simulink model "N3_TE0722A4"  (R2013b)
settings: Solver=ode45  StartTime=0.0  StopTime=1e-4  RelTol=1e-3
PreLoadFcn:
  | fpgaclk=1/32.768e6
  | SerialData=[1,zeros(1,11),1,0,0,1]
  | load ../window
  | win=win'   %Go back to using flatter and wider windowed sync function
  | %load ../hanning    %use Hahn window
  | 
  | load ../PREemphasis   %For pre-empasis and deemphasis FIRs
  | 
  | LUT3=xls2LUT2('../IQI_Qdemod.xls')
  | load ../FIRiq2
  | % xls2LUT
  | 
  | GetProgFiles
  | 
  | PinAssignments    %Get Pin references for TE0722
  | 
  | 
  | 
  | 
  | 
  | %LCD
  | LCDdata=[LCD_D7,LCD_D6,LCD_D5,LCD_D4,LCD_D3,LCD_D2,LCD_D1,LCD_D0] %Note MSB...LSB!
  | LCDctrl=[LCD_E,LCD_RW,LCD_RS];
  | 
  | %for RS232 on pins 3 and 5 of USBB
  | 
  | %BT chip connections for WT12
  | 
  | RX_BT=RXD
  | TX_BT=TXD
  | 
  | RST_BB=RES
  | 
  | %PCMC=PCMC
  | %PCMS=PCMS
  | %PCMI=PCMI
  | %PCMO=PCMO
  | 
  | %Aliases:
  | SRDBT=PCMI
  | STDBT=PCMO
  | SCLK_BT=PCMC
  | SFS_BT=PCMS
  | 
  | %ADC control
  | 
  | %SDOA=SDOA
  | %SDOB=SDOB
  | %SCK=SCK
  | CONV=Csbar
  | CAL=Cal
  | 
  | ADC_G=[ADC_G3,ADC_G2,ADC_G1,ADC_G0]
  | %PD settings hard coded now
  | 
  | %%%%%%
  | TX_LOW=TX_Low
  | 
  | %Leds
  | %Defined inPinassignments
  | ... (+8 lines)
StartFcn:
  | fpgaclk=1/32.768e6
  | SerialData=[1,zeros(1,11),1,0,0,1]
values from neighbouring files (symbols this model uses):
  ADC_G0 = {'P10'}    [PinAssignments.m]
  ADC_G1 = {'P11'}    [PinAssignments.m]
  ADC_G2 = {'N14'}    [PinAssignments.m]
  ADC_G3 = {'M11'}    [PinAssignments.m]
  Cal = {'L12'}    [PinAssignments.m]
  Csbar = {'M12'}    [PinAssignments.m]
  LCD_D0 = {'J13'}    [PinAssignments.m]
  LCD_D1 = {'J14'}    [PinAssignments.m]
  LCD_D2 = {'F15'}    [PinAssignments.m]
  LCD_D3 = {'H14'}    [PinAssignments.m]
  LCD_D4 = {'G12'}    [PinAssignments.m]
  LCD_D5 = {'L15'}    [PinAssignments.m]
  LCD_D6 = {'M14'}    [PinAssignments.m]
  LCD_D7 = {'K15'}    [PinAssignments.m]
  PCMC = {'H11'}    [PinAssignments.m]
  PCMI = {'H12'}    [PinAssignments.m]
  PCMO = {'N13'}    [PinAssignments.m]
  PCMS = {'M10'}    [PinAssignments.m]
  RES = {'G11'}    [PinAssignments.m]
  RXD = {'H13'}    [PinAssignments.m]
  TX_Low = {'P15'}    [PinAssignments.m]
  TXD = {'P13'}    [PinAssignments.m]
undefined symbols (not defined in the file or in its folder): FIRRX, FIRTX
libraries: xbsIndex_r4 x1100, MyFunctions x42
(part 2 of 9)

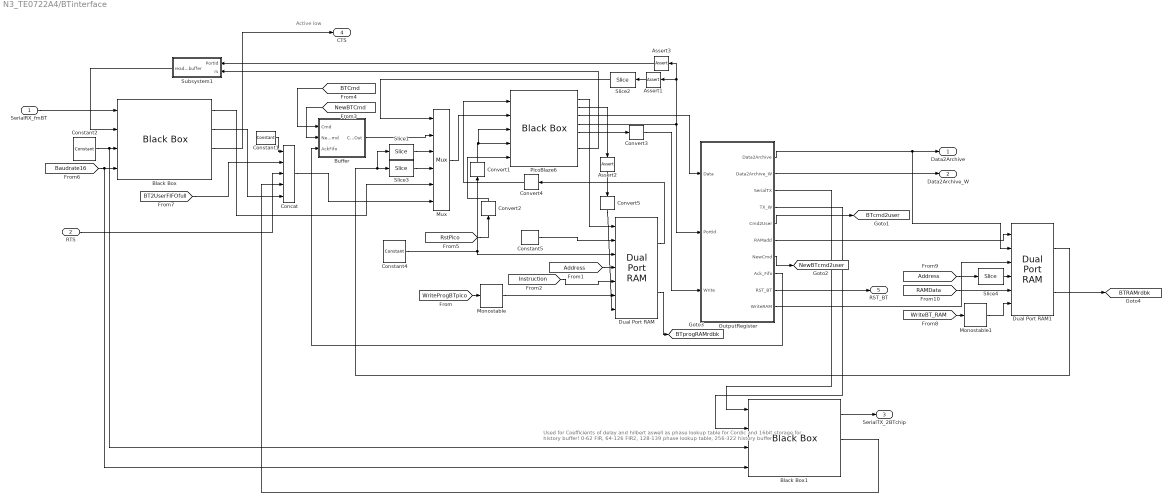
== system N3_TE0722A4/BTinterface ==
  note: Used for Coefficients of delay and hilbert aswell as phase lookup table for Cordic and 16bit storage for history buffer!
      | 0-62 FIR, 64-126 FIR2, 128-139 phase lookup table, 256-322 history buffer
  note: Active low
  SerialRX_fmBT : Inport
  RTS : Inport  Port=2
  Assert1 : xbsIndex_r4/Assert  assert_type=off  type_source=Explicitly  gui_display_data_type=Fixed-point  arith_type="Signed  (2's comp)"  n_bits=16  bin_pt=14  preci_type=Single  exp_width=8  frac_width=24  assert_rate=on  rate_source=Explicitly  period=fpgaclk  output_port=on  block_type=assert
  Assert2 : xbsIndex_r4/Assert  assert_type=off  type_source=Explicitly  gui_display_data_type=Fixed-point  arith_type="Signed  (2's comp)"  n_bits=16  bin_pt=14  preci_type=Single  exp_width=8  frac_width=24  assert_rate=on  rate_source=Explicitly  period=fpgaclk  output_port=on  block_type=assert
  Assert3 : xbsIndex_r4/Assert  assert_type=off  type_source=Explicitly  gui_display_data_type=Fixed-point  arith_type="Signed  (2's comp)"  n_bits=16  bin_pt=14  preci_type=Single  exp_width=8  frac_width=24  assert_rate=on  rate_source=Explicitly  period=fpgaclk  output_port=on  block_type=assert
  Black Box : xbsIndex_r4/Black Box  init_code=uart_rxce_config  sim_method=Inactive  verbose=off  block_type=blackbox2
      settings: block_version=8.2.02
  Black Box1 : xbsIndex_r4/Black Box  init_code=uart_txce_config  sim_method=Inactive  verbose=off  block_type=blackbox2
      settings: infoedit="Incorporates black box HDL and simulation model into a System Generator design.<P><P>You must supply a Black Box with certain information about the HDL component you would like to bring into System Generator. This information is provided through a Matlab function.<P><P>When \"Simulation mode\" is set to \"Inactive\", you will typically want to provide a separate simulation model by using a Simulation Multiplexer.<P>When \"Simulation mode\" is set to \"External co-simulator\", you must include a ModelSim block in the design."  block_version=8.2.02
  Buffer : Subsystem
  Concat : xbsIndex_r4/Concat  num_inputs=5  dbl_ovrd=off  block_type=concat
      settings: block_version=VER_STRING_GOES_HERE
  Constant1 : xbsIndex_r4/Constant  const=0  gui_display_data_type=Fixed-point  arith_type=Unsigned  n_bits=4  bin_pt=0  preci_type=Single  exp_width=8  frac_width=24  explicit_period=on  period=fpgaclk  equ=P=C  opselect=C  inp2=PCIN>>17  opr=+  inp1=P  carry=CIN  dbl_ovrd=off  block_type=constant
      settings: block_version=VER_STRING_GOES_HERE
  Constant2 : xbsIndex_r4/Constant  const=0  gui_display_data_type=Fixed-point  arith_type=Unsigned  n_bits=1  bin_pt=0  preci_type=Single  exp_width=8  frac_width=24  explicit_period=on  period=fpgaclk  equ=P=C  opselect=C  inp2=PCIN>>17  opr=+  inp1=P  carry=CIN  dbl_ovrd=off  block_type=constant
      settings: block_version=VER_STRING_GOES_HERE
  Constant4 : xbsIndex_r4/Constant  const=0  gui_display_data_type=Fixed-point  arith_type=Boolean  n_bits=1  bin_pt=0  preci_type=Single  exp_width=8  frac_width=24  explicit_period=on  period=fpgaclk  equ=P=C  opselect=C  inp2=PCIN>>17  opr=+  inp1=P  carry=CIN  dbl_ovrd=off  block_type=constant
      settings: block_version=VER_STRING_GOES_HERE
  Constant5 : xbsIndex_r4/Constant  const=0  gui_display_data_type=Fixed-point  arith_type=Unsigned  n_bits=18  bin_pt=0  preci_type=Single  exp_width=8  frac_width=24  explicit_period=on  period=fpgaclk  equ=P=C  opselect=C  inp2=PCIN>>17  opr=+  inp1=P  carry=CIN  dbl_ovrd=off  block_type=constant
      settings: block_version=VER_STRING_GOES_HERE
  Convert1 : xbsIndex_r4/Convert  gui_display_data_type=Fixed-point  arith_type=Boolean  n_bits=16  bin_pt=0  float_type=Single  exp_bits=8  fraction_bits=24  quantization=Truncate  overflow=Wrap  en=off  latency=0  pipeline=off  dbl_ovrd=off  block_type=convert
      settings: xl_area=[0 0 0 0 0 0 0]  block_version=VER_STRING_GOES_HERE
  Convert2 : xbsIndex_r4/Convert  gui_display_data_type=Fixed-point  arith_type=Boolean  n_bits=16  bin_pt=0  float_type=Single  exp_bits=8  fraction_bits=24  quantization=Truncate  overflow=Wrap  en=off  latency=0  pipeline=off  dbl_ovrd=off  block_type=convert
      settings: xl_area=[0, 0, 0, 0, 0, 0, 0]  block_version=VER_STRING_GOES_HERE
  Convert3 : xbsIndex_r4/Convert  gui_display_data_type=Fixed-point  arith_type=Boolean  n_bits=16  bin_pt=0  float_type=Single  exp_bits=8  fraction_bits=24  quantization=Truncate  overflow=Wrap  en=off  latency=0  pipeline=off  dbl_ovrd=off  block_type=convert
      settings: xl_area=[0 0 0 0 0 0 0]  block_version=VER_STRING_GOES_HERE
  Convert4 : xbsIndex_r4/Convert  gui_display_data_type=Fixed-point  arith_type=Unsigned  n_bits=18  bin_pt=0  float_type=Single  exp_bits=8  fraction_bits=24  quantization=Truncate  overflow=Wrap  en=off  latency=0  pipeline=off  dbl_ovrd=off  block_type=convert
      settings: xl_area=[0, 0, 0, 0, 0, 0, 0]  block_version=VER_STRING_GOES_HERE
  Convert5 : xbsIndex_r4/Convert  gui_display_data_type=Boolean  arith_type=Boolean  n_bits=18  bin_pt=0  float_type=Single  exp_bits=8  fraction_bits=24  quantization=Truncate  overflow=Wrap  en=off  latency=0  pipeline=off  dbl_ovrd=off  block_type=convert
      settings: xl_area=[0, 0, 0, 0, 0, 0, 0]  block_version=VER_STRING_GOES_HERE
  Dual Port RAM : xbsIndex_r4/Dual Port RAM  depth=1024*4  initVector=BTprog  distributed_mem=Block RAM  init_a=0  init_b=0  rst_a=off  rst_b=off  en_a=on  en_b=off  latency=1  write_mode_A=Read After Write  write_mode_B=Read After Write  optimize=Area  dbl_ovrd=off  block_type=dpram
      settings: block_version=8.2.02
  Dual Port RAM1 : xbsIndex_r4/Dual Port RAM  depth=1024  initVector=BTmessages  distributed_mem=Block RAM  init_a=0  init_b=0  rst_a=off  rst_b=off  en_a=off  en_b=off  latency=1  write_mode_A=Read After Write  write_mode_B=Read After Write  optimize=Area  dbl_ovrd=off  block_type=dpram
      settings: block_version=8.2.02
  Monostable : MyFunctions/Monostable
  Monostable1 : MyFunctions/Monostable
  Mux : xbsIndex_r4/Mux  inputs=5  en=off  latency=1  precision=Full  arith_type=Unsigned  n_bits=16  bin_pt=14  quantization=Truncate  overflow=Wrap  dbl_ovrd=off  block_type=mux
      settings: xl_area=[16 0 0 32 0 0 0]  block_version=VER_STRING_GOES_HERE
  OutputRegister : Subsystem
  PicoBlaze6 : xbsIndex_r4/Black Box  init_code=kcpsm6_CE_256_4k_config  sim_method=Inactive  verbose=off  block_type=blackbox2
  Slice1 : xbsIndex_r4/Slice  nbits=8  boolean_output=off  mode=Lower Bit Location + Width  bit1=0  base1=MSB of Input  bit0=8  base0=LSB of Input  dbl_ovrd=off  block_type=slice
      settings: block_version=VER_STRING_GOES_HERE
  Slice2 : xbsIndex_r4/Slice  nbits=3  boolean_output=off  mode=Lower Bit Location + Width  bit1=0  base1=MSB of Input  bit0=0  base0=LSB of Input  dbl_ovrd=off  block_type=slice
      settings: block_version=VER_STRING_GOES_HERE
  Slice3 : xbsIndex_r4/Slice  nbits=8  boolean_output=off  mode=Lower Bit Location + Width  bit1=0  base1=MSB of Input  bit0=0  base0=LSB of Input  dbl_ovrd=off  block_type=slice
      settings: block_version=VER_STRING_GOES_HERE
  Slice4 : xbsIndex_r4/Slice  nbits=10  boolean_output=off  mode=Lower Bit Location + Width  bit1=0  base1=MSB of Input  bit0=0  base0=LSB of Input  dbl_ovrd=off  block_type=slice
      settings: block_version=VER_STRING_GOES_HERE
  Subsystem1 : Subsystem
  Data2Archive : Outport
  Data2Archive_W : Outport  Port=2
  SerialTX_2BTchip : Outport  Port=3
  CTS : Outport  Port=4
  RST_BT : Outport  Port=5
  tag scope: BTRAMrdbk=global, BTcmd2user=global, BTprogRAMrdbk=global, NewBTcmd2user=global
  wires:
  Convert4/1 -> PicoBlaze6/1
  [RstPico] -> Convert2/1
  PicoBlaze6/5 -> Convert3/1
  PicoBlaze6/4 -> Assert1/1, Assert3/1, OutputRegister/2(PortId)
  PicoBlaze6/3 -> OutputRegister/1(Data)
  PicoBlaze6/1 -> Dual Port RAM/1
  Convert2/1 -> PicoBlaze6/5
  Mux/1 -> PicoBlaze6/2
  Dual Port RAM/1 -> Convert4/1
  Constant4/1 -> Dual Port RAM/3, Convert1/1
  Constant5/1 -> Dual Port RAM/2
  Slice2/1 -> Mux/1
  Convert1/1 -> PicoBlaze6/3, PicoBlaze6/4
  OutputRegister/5(Cmd2User) -> [BTcmd2user]
  OutputRegister/8(Ack_Fifo) -> Buffer/3(AckFifo)
  Convert3/1 -> OutputRegister/3(Write)
  OutputRegister/1(Data2Archive) -> Data2Archive/1, Dual Port RAM1/2
  [Address] -> Dual Port RAM/4
  Buffer/1(CmdOut) -> Mux/2
  [Instruction] -> Dual Port RAM/5
  OutputRegister/7(NewCmd) -> [NewBTcmd2user]
  [BTCmd] -> Buffer/1(Cmd)
  [NewBTCmd] -> Buffer/2(NewCmd)
  Black Box/1 -> Mux/5
  Subsystem1/1(read_buffer) -> Black Box/2
  Constant1/1 -> Concat/1
  PicoBlaze6/7 -> Subsystem1/2(rs)
  Black Box1/1 -> SerialTX_2BTchip/1
  Black Box/2 -> Concat/5
  Concat/1 -> Mux/6
  SerialRX_fmBT/1 -> Black Box/1
  RTS/1 -> Concat/3
  Black Box/3 -> CTS/1
  OutputRegister/3(SerialTX) -> Black Box1/1
  OutputRegister/4(TX_W) -> Black Box1/2
  [Baudrate16] -> Black Box/4, Black Box1/4
  OutputRegister/2(Data2Archive_W) -> Data2Archive_W/1
  OutputRegister/9(RST_BT) -> RST_BT/1
  Monostable/1 -> Dual Port RAM/6
  Constant2/1 -> Black Box/3, Black Box1/3
  [BT2UserFIFOfull] -> Concat/2
  Black Box1/2 -> Concat/4
  [WriteProgBTpico] -> Monostable/1
  Dual Port RAM/2 -> [BTprogRAMrdbk]
  [Address] -> Slice4/1
  [RAMData] -> Dual Port RAM1/5
  Monostable1/1 -> Dual Port RAM1/6
  [WriteBT_RAM] -> Monostable1/1
  Dual Port RAM1/2 -> [BTRAMrdbk]
  OutputRegister/6(RAMadd) -> Dual Port RAM1/1
  Slice1/1 -> Mux/3
  Slice3/1 -> Mux/4
  Dual Port RAM1/1 -> Slice1/1, Slice3/1
  OutputRegister/10(WriteRAM) -> Dual Port RAM1/3
  Slice4/1 -> Dual Port RAM1/4
  PicoBlaze6/2 -> Assert2/1
  Assert3/1 -> Subsystem1/1(PortId)
  Assert1/1 -> Slice2/1
  Assert2/1 -> Convert5/1
  Convert5/1 -> Dual Port RAM/7

== system N3_TE0722A4/Bit_Corrector ==
  note: Does the sign extnsion
  In1 : Inport
  Concat : xbsIndex_r4/Concat  num_inputs=3  dbl_ovrd=off  block_type=concat
      settings: block_version=12.2
  Reinterpret : xbsIndex_r4/Reinterpret  force_arith_type=on  arith_type="Signed  (2's comp)"  force_bin_pt=on  bin_pt=15  block_type=reinterpret
      settings: infoedit="Changes signal type without altering the binary representation.   You can changed the signal between signed and unsigned, and relocate the binary point.<br><br>Hardware notes: In hardware this block costs nothing.<br><br>Example:  Suppose the input is 6 bits wide, signed, with 2 fractional bits, and the output is forced to unsigned with 0 fractional bits.  Then an input of -2.0 (1110.00 in binary 2's complement) becomes an output of 56 (111000 in binary)."  block_version=8.2.02
  Slice : xbsIndex_r4/Slice  nbits=14  boolean_output=off  mode=Lower Bit Location + Width  bit1=0  base1=MSB of Input  bit0=0  base0=LSB of Input  dbl_ovrd=off  block_type=slice
      settings: block_version=12.2
  Slice1 : xbsIndex_r4/Slice  nbits=1  boolean_output=off  mode=Lower Bit Location + Width  bit1=0  base1=MSB of Input  bit0=13  base0=LSB of Input  dbl_ovrd=off  block_type=slice
      settings: block_version=12.2
  Slice2 : xbsIndex_r4/Slice  nbits=1  boolean_output=off  mode=Lower Bit Location + Width  bit1=0  base1=MSB of Input  bit0=13  base0=LSB of Input  dbl_ovrd=off  block_type=slice
      settings: block_version=12.2
  Out1 : Outport
  wires:
  In1/1 -> Slice2/1, Slice1/1, Slice/1
  Slice2/1 -> Concat/1
  Slice1/1 -> Concat/2
  Slice/1 -> Concat/3
  Concat/1 -> Reinterpret/1
  Reinterpret/1 -> Out1/1

== system N3_TE0722A4/Bit_Corrector1 ==
  note: Does the sign extnsion
  In1 : Inport
  Concat : xbsIndex_r4/Concat  num_inputs=3  dbl_ovrd=off  block_type=concat
      settings: block_version=12.2
  Reinterpret : xbsIndex_r4/Reinterpret  force_arith_type=on  arith_type="Signed  (2's comp)"  force_bin_pt=on  bin_pt=15  block_type=reinterpret
      settings: infoedit="Changes signal type without altering the binary representation.   You can changed the signal between signed and unsigned, and relocate the binary point.<br><br>Hardware notes: In hardware this block costs nothing.<br><br>Example:  Suppose the input is 6 bits wide, signed, with 2 fractional bits, and the output is forced to unsigned with 0 fractional bits.  Then an input of -2.0 (1110.00 in binary 2's complement) becomes an output of 56 (111000 in binary)."  block_version=8.2.02
  Slice : xbsIndex_r4/Slice  nbits=14  boolean_output=off  mode=Lower Bit Location + Width  bit1=0  base1=MSB of Input  bit0=0  base0=LSB of Input  dbl_ovrd=off  block_type=slice
      settings: block_version=12.2
  Slice1 : xbsIndex_r4/Slice  nbits=1  boolean_output=off  mode=Lower Bit Location + Width  bit1=0  base1=MSB of Input  bit0=13  base0=LSB of Input  dbl_ovrd=off  block_type=slice
      settings: block_version=12.2
  Slice2 : xbsIndex_r4/Slice  nbits=1  boolean_output=off  mode=Lower Bit Location + Width  bit1=0  base1=MSB of Input  bit0=13  base0=LSB of Input  dbl_ovrd=off  block_type=slice
      settings: block_version=12.2
  Out1 : Outport
  wires:
  In1/1 -> Slice2/1, Slice1/1, Slice/1
  Slice2/1 -> Concat/1
  Slice1/1 -> Concat/2
  Slice/1 -> Concat/3
  Concat/1 -> Reinterpret/1
  Reinterpret/1 -> Out1/1

== system N3_TE0722A4/ConstantDetect ==
  note: Pulses every 8 pulses of the 8kHz strobe ie at 1kHz
  Signal : Inport
  Strobe : Inport  Port=2
  Constant1 : xbsIndex_r4/Constant  const=4  gui_display_data_type=Fixed-point  arith_type=Unsigned  n_bits=4  bin_pt=0  preci_type=Single  exp_width=8  frac_width=24  explicit_period=off  period=1  equ=P=C  opselect=C  inp2=PCIN>>17  opr=+  inp1=P  carry=CIN  dbl_ovrd=off  block_type=constant
      settings: block_version=12.2
  Convert : xbsIndex_r4/Convert  gui_display_data_type=Fixed-point  arith_type=Boolean  n_bits=16  bin_pt=14  float_type=Single  exp_bits=8  fraction_bits=24  quantization=Truncate  overflow=Wrap  en=off  latency=0  pipeline=off  dbl_ovrd=off  block_type=convert
      settings: block_version=12.2
  Counter : xbsIndex_r4/Counter  cnt_type=Free Running  cnt_to=Inf  operation=Up  start_count=0  cnt_by_val=1  arith_type=Unsigned  n_bits=3  bin_pt=0  load_pin=off  rst=off  en=on  explicit_period=on  period=fpgaclk  use_behavioral_HDL=off  implementation=Fabric  dbl_ovrd=off  block_type=counter
      settings: block_version=12.2
  Counter1 : xbsIndex_r4/Counter  cnt_type=Free Running  cnt_to=Inf  operation=Up  start_count=0  cnt_by_val=1  arith_type=Unsigned  n_bits=4  bin_pt=0  load_pin=off  rst=on  en=on  explicit_period=on  period=fpgaclk  use_behavioral_HDL=off  implementation=Fabric  dbl_ovrd=off  block_type=counter
      settings: block_version=12.2
  Delay : xbsIndex_r4/Delay  rst=off  infoeditControl=Selection of Reset will increase slice count due to use of real FFs and instead of SRLs  en=on  latency=1  reg_retiming=off  dbl_ovrd=off  block_type=delay
      settings: block_version=12.2
  Delay1 : xbsIndex_r4/Delay  rst=off  infoeditControl=Selection of Reset will increase slice count due to use of real FFs and instead of SRLs  en=on  latency=1  reg_retiming=off  dbl_ovrd=off  block_type=delay
      settings: block_version=12.2
  Logical : xbsIndex_r4/Logical  logical_function=AND  inputs=2  en=off  latency=0  precision=Full  arith_type=Unsigned  n_bits=16  bin_pt=0  align_bp=on  dbl_ovrd=off  block_type=logical
      settings: block_version=12.2
  Monostable : MyFunctions/Monostable
  Register : xbsIndex_r4/Register  init=0  rst=off  en=on  dbl_ovrd=off  block_type=register
      settings: block_version=12.2
  Relational : xbsIndex_r4/Relational  mode=a=b  op_type=Bool  en=off  latency=1  dbl_ovrd=off  block_type=relational
      settings: block_version=12.2
  Relational1 : xbsIndex_r4/Relational  mode=a<b  op_type=Bool  en=off  latency=1  dbl_ovrd=off  block_type=relational
      settings: block_version=12.2
  Slice : xbsIndex_r4/Slice  nbits=1  boolean_output=off  mode=Upper Bit Location + Width  bit1=0  base1=MSB of Input  bit0=0  base0=LSB of Input  dbl_ovrd=off  block_type=slice
      settings: block_version=12.2
  IsConstant : Outport
  wires:
  Signal/1 -> Delay/1
  Strobe/1 -> Delay/2, Delay1/2, Counter/1, Logical/2
  Counter/1 -> Slice/1
  Slice/1 -> Convert/1
  Convert/1 -> Monostable/1
  Monostable/1 -> Counter1/1, Register/2
  Counter1/1 -> Register/1
  Constant1/1 -> Relational1/1
  Register/1 -> Relational1/2
  Relational1/1 -> IsConstant/1
  Relational/1 -> Logical/1
  Logical/1 -> Counter1/2
  Delay/1 -> Delay1/1, Relational/1
  Delay1/1 -> Relational/2

== system N3_TE0722A4/DAC (XAPP154) ==
  note: This subsystem implements a delta-sigma DAC
  note: The 'Delta Adder' computes the difference
      | between the current DAC input and the current
      | DAC output.  The two concatenators create
      | a 16-bit output with the DAC output copied in the
      | two MSB positions. This effectively creates a
      | difference from the 'Delta Adder' when the DAC
      | output is 1.
  note: The 'Sigma Adder' accumulates the
      | differences produced by the 'Delta Adder'
      | by using 'r1' to storing the adder output on
      | each succesive cycle.  The MSB of the 'r1'
      | output is sliced off and provides the DAC
      | output.
  note: The pulse string is registered before
      | it is driven on the DAC output port.
  note: Constants sampled at 40*fpgaclk
      | to reduce modulation frequency
  DAC_In : Inport
  Disable_Audio : Inport  Port=2
  Concat : xbsIndex_r4/Concat  num_inputs=2  dbl_ovrd=off  block_type=concat
      settings: block_version=VER_STRING_GOES_HERE
  Concat1 : xbsIndex_r4/Concat  num_inputs=2  dbl_ovrd=off  block_type=concat
      settings: block_version=VER_STRING_GOES_HERE
  Constant : xbsIndex_r4/Constant  const=0  gui_display_data_type=Fixed-point  arith_type=Boolean  n_bits=1  bin_pt=0  preci_type=Single  exp_width=8  frac_width=24  explicit_period=on  period=fpgaclk*40  equ=P=C  opselect=C  inp2=PCIN>>17  opr=+  inp1=P  carry=CIN  dbl_ovrd=off  block_type=constant
      settings: block_version=VER_STRING_GOES_HERE
  Constant2 : xbsIndex_r4/Constant  const=0  gui_display_data_type=Fixed-point  arith_type=Unsigned  n_bits=14  bin_pt=0  preci_type=Single  exp_width=8  frac_width=24  explicit_period=on  period=fpgaclk*40  equ=P=C  opselect=C  inp2=PCIN>>17  opr=+  inp1=P  carry=CIN  dbl_ovrd=off  block_type=constant
      settings: block_version=VER_STRING_GOES_HERE
  Delta Adder : xbsIndex_r4/AddSub  mode=Addition  use_carryin=off  use_carryout=off  en=on  latency=1  precision=User Defined  arith_type=Unsigned  n_bits=16  bin_pt=0  quantization=Truncate  overflow=Wrap  use_behavioral_HDL=on  hw_selection=Fabric  pipelined=off  use_rpm=off  dbl_ovrd=off  block_type=addsub
      settings: xl_area=[8 0 0 16 0 0 0]  block_version=VER_STRING_GOES_HERE
  Inverter : xbsIndex_r4/Inverter  en=off  latency=0  dbl_ovrd=off  block_type=inv
      settings: block_version=8.2.02
  Register1 : xbsIndex_r4/Register  init=0  rst=on  en=off  dbl_ovrd=off  block_type=register
      settings: xl_area=[1 1 0 0 0 0 0]  block_version=VER_STRING_GOES_HERE
  Sigma Adder : xbsIndex_r4/AddSub  mode=Addition  use_carryin=off  use_carryout=off  en=off  latency=0  precision=User Defined  arith_type=Unsigned  n_bits=16  bin_pt=0  quantization=Truncate  overflow=Wrap  use_behavioral_HDL=on  hw_selection=Fabric  pipelined=off  use_rpm=off  dbl_ovrd=off  block_type=addsub
      settings: xl_area=[8 0 0 16 0 0 0]  block_version=VER_STRING_GOES_HERE
  Slice1 : xbsIndex_r4/Slice  nbits=1  boolean_output=off  mode=Upper Bit Location + Width  bit1=0  base1=MSB of Input  bit0=0  base0=LSB of Input  dbl_ovrd=off  block_type=slice
      settings: infoedit="Extracts a given range of bits from each input sample and presents it at the output.  The output type is ordinarily unsigned with binary point at zero, but can be Boolean when the slice is one bit wide.<P><P>Hardware notes: In hardware this block costs nothing."  block_version=VER_STRING_GOES_HERE
  r1 : xbsIndex_r4/Register  init=2^6  rst=on  en=off  dbl_ovrd=off  block_type=register
      settings: xl_area=[8 16 0 0 0 0 0]  block_version=VER_STRING_GOES_HERE
  DAC_Out : Outport
  wires:
  DAC_In/1 -> Delta Adder/1
  Register1/1 -> DAC_Out/1
  r1/1 -> Slice1/1, Sigma Adder/1
  Sigma Adder/1 -> r1/1
  Constant/1 -> r1/2
  Concat1/1 -> Delta Adder/2
  Concat/1 -> Concat1/1
  Slice1/1 -> Register1/1, Concat/1, Concat/2
  Constant2/1 -> Concat1/2
  Delta Adder/1 -> Sigma Adder/2
  Disable_Audio/1 -> Register1/2, Inverter/1
  Inverter/1 -> Delta Adder/3

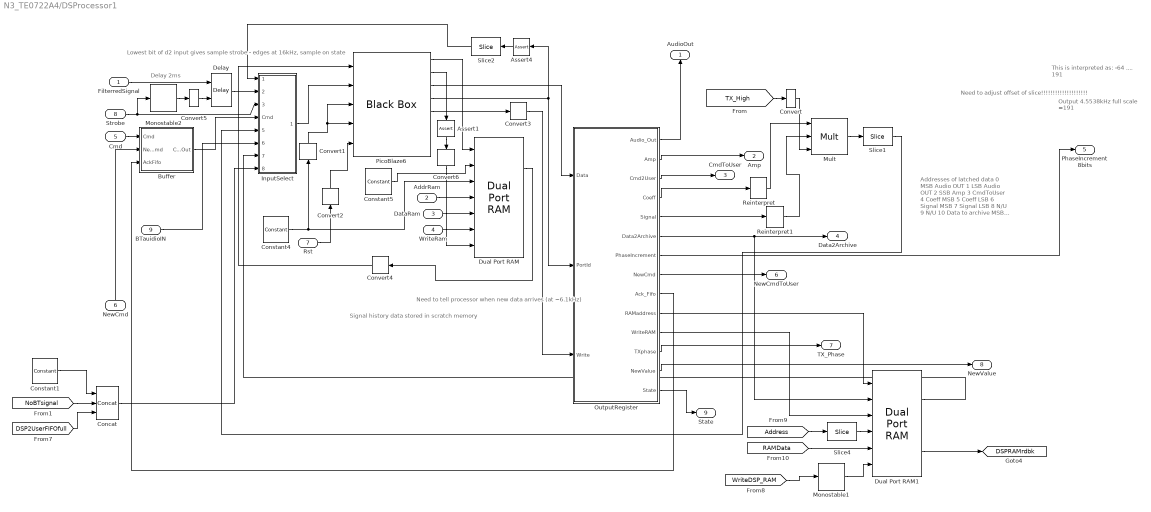
== system N3_TE0722A4/DSProcessor1 ==
  note: Need to adjust offset of slice!!!!!!!!!!!!!!!!!!!!
  note: Need to tell processor when new data arrives (at ~6.1kHz)
  note: Lowest bit of d2 input gives sample strobe - edges at 16kHz, sample on state
  note: Output 4.5538kHz
      | full scale =191
  note: This is interpreted as:
      | -64 .... 191
  note: Signal history data stored in scratch memory
  note: Addresses of latched data
      | 0 MSB Audio OUT
      | 1 LSB Audio OUT
      | 2 SSB Amp
      | 3 CmdToUser
      | 4 Coeff MSB
      | 5 Coeff LSB
      | 6 Signal MSB
      | 7 Signal LSB
      | 8 N/U
      | 9 N/U
      | 10 Data to archive MSB
      | 11 Data to archive LSB
      | 12 Control bits:
      | 	0
      | 	1
      | 	2
      | 	3
      | 	4
      | 	5 Ack Fifo
      |
      | 13 Audio Freq MSB
  note: Delay 2ms
  FilterredSignal : Inport
  AddrRam : Inport  Port=2
  DataRam : Inport  Port=3
  WriteRam : Inport  Port=4
  Cmd : Inport  Port=5
  NewCmd : Inport  Port=6
  Rst : Inport  Port=7
  Strobe : Inport  Port=8
  BTauidioIN : Inport  Port=9
  Assert1 : xbsIndex_r4/Assert  assert_type=off  type_source=Explicitly  gui_display_data_type=Fixed-point  arith_type="Signed  (2's comp)"  n_bits=16  bin_pt=14  preci_type=Single  exp_width=8  frac_width=24  assert_rate=on  rate_source=Explicitly  period=fpgaclk  output_port=on  block_type=assert
  Assert4 : xbsIndex_r4/Assert  assert_type=off  type_source=Explicitly  gui_display_data_type=Fixed-point  arith_type="Signed  (2's comp)"  n_bits=16  bin_pt=14  preci_type=Single  exp_width=8  frac_width=24  assert_rate=on  rate_source=Explicitly  period=fpgaclk  output_port=on  block_type=assert
  Buffer : Subsystem
  Concat : xbsIndex_r4/Concat  num_inputs=3  dbl_ovrd=off  block_type=concat
      settings: block_version=12.2
  Constant1 : xbsIndex_r4/Constant  const=0  gui_display_data_type=Fixed-point  arith_type=Unsigned  n_bits=6  bin_pt=0  preci_type=Single  exp_width=8  frac_width=24  explicit_period=on  period=fpgaclk  equ=P=C  opselect=C  inp2=PCIN>>17  opr=+  inp1=P  carry=CIN  dbl_ovrd=off  block_type=constant
      settings: block_version=VER_STRING_GOES_HERE
  Constant4 : xbsIndex_r4/Constant  const=0  gui_display_data_type=Fixed-point  arith_type=Boolean  n_bits=1  bin_pt=0  preci_type=Single  exp_width=8  frac_width=24  explicit_period=on  period=fpgaclk  equ=P=C  opselect=C  inp2=PCIN>>17  opr=+  inp1=P  carry=CIN  dbl_ovrd=off  block_type=constant
      settings: block_version=VER_STRING_GOES_HERE
  Constant5 : xbsIndex_r4/Constant  const=0  gui_display_data_type=Fixed-point  arith_type=Unsigned  n_bits=18  bin_pt=0  preci_type=Single  exp_width=8  frac_width=24  explicit_period=on  period=fpgaclk  equ=P=C  opselect=C  inp2=PCIN>>17  opr=+  inp1=P  carry=CIN  dbl_ovrd=off  block_type=constant
      settings: block_version=VER_STRING_GOES_HERE
  Convert : xbsIndex_r4/Convert  gui_display_data_type=Fixed-point  arith_type=Boolean  n_bits=16  bin_pt=14  float_type=Single  exp_bits=8  fraction_bits=24  quantization=Truncate  overflow=Wrap  en=off  latency=0  pipeline=off  dbl_ovrd=off  block_type=convert
      settings: block_version=8.2.02
  Convert{1..3,5..6} (5 alike) : xbsIndex_r4/Convert  gui_display_data_type=Fixed-point  arith_type=Boolean  n_bits=16  bin_pt=0  float_type=Single  exp_bits=8  fraction_bits=24  quantization=Truncate  overflow=Wrap  en=off  latency=0  pipeline=off  dbl_ovrd=off  block_type=convert
      Convert1 settings: xl_area=[0 0 0 0 0 0 0]  block_version=VER_STRING_GOES_HERE
      Convert2 settings: xl_area=[0, 0, 0, 0, 0, 0, 0]  block_version=VER_STRING_GOES_HERE
      Convert3 settings: xl_area=[0 0 0 0 0 0 0]  block_version=VER_STRING_GOES_HERE
      Convert5 settings: xl_area=[0 0 0 0 0 0 0]  block_version=VER_STRING_GOES_HERE
      Convert6 settings: xl_area=[0 0 0 0 0 0 0]  block_version=VER_STRING_GOES_HERE
  Convert4 : xbsIndex_r4/Convert  gui_display_data_type=Fixed-point  arith_type=Unsigned  n_bits=18  bin_pt=0  float_type=Single  exp_bits=8  fraction_bits=24  quantization=Truncate  overflow=Wrap  en=off  latency=0  pipeline=off  dbl_ovrd=off  block_type=convert
      settings: xl_area=[0, 0, 0, 0, 0, 0, 0]  block_version=VER_STRING_GOES_HERE
  Delay : xbsIndex_r4/Delay  rst=off  infoeditControl=Selection of Reset will increase slice count due to use of real FFs and instead of SRLs  en=on  latency=17  reg_retiming=off  dbl_ovrd=off  block_type=delay
      settings: block_version=12.2
  Dual Port RAM : xbsIndex_r4/Dual Port RAM  depth=1024*4  initVector=DSPprog  distributed_mem=Block RAM  init_a=0  init_b=0  rst_a=off  rst_b=off  en_a=on  en_b=off  latency=1  write_mode_A=Read After Write  write_mode_B=Read After Write  optimize=Area  dbl_ovrd=off  block_type=dpram
      settings: block_version=8.2.02
  Dual Port RAM1 : xbsIndex_r4/Dual Port RAM  depth=1024  initVector=zeros(1024,1)  distributed_mem=Block RAM  init_a=0  init_b=0  rst_a=off  rst_b=off  en_a=off  en_b=off  latency=1  write_mode_A=Read After Write  write_mode_B=Read After Write  optimize=Area  dbl_ovrd=off  block_type=dpram
      settings: block_version=8.2.02
  InputSelect : Subsystem
  Monostable1 : MyFunctions/Monostable
  Monostable2 : MyFunctions/Monostable
  Mult : xbsIndex_r4/Mult  precision=Full  arith_type="Signed  (2's comp)"  n_bits=16  bin_pt=14  quantization=Truncate  overflow=Wrap  en=on  latency=3  use_behavioral_HDL=off  opt=Speed  use_embedded=on  optimum_pipeline=off  pipeline=on  dbl_ovrd=off  use_rpm=on  placement_style=Rectangular shape  block_type=mult
      settings: infoedit=Hardware notes: To use the internal pipeline stage of the dedicated multiplier you must select 'Pipeline for maximum performance'.  block_version=8.2.02
  OutputRegister : Subsystem
  PicoBlaze6 : xbsIndex_r4/Black Box  init_code=kcpsm6_CE_256_4k_config  sim_method=Inactive  verbose=off  block_type=blackbox2
  Reinterpret : xbsIndex_r4/Reinterpret  force_arith_type=on  arith_type="Signed  (2's comp)"  force_bin_pt=off  bin_pt=0  block_type=reinterpret
  Reinterpret1 : xbsIndex_r4/Reinterpret  force_arith_type=on  arith_type="Signed  (2's comp)"  force_bin_pt=off  bin_pt=0  block_type=reinterpret
  Slice1 : xbsIndex_r4/Slice  nbits=24  boolean_output=off  mode=Upper Bit Location + Width  bit1=0  base1=MSB of Input  bit0=0  base0=LSB of Input  dbl_ovrd=off  block_type=slice
      settings: block_version=VER_STRING_GOES_HERE
  Slice2 : xbsIndex_r4/Slice  nbits=4  boolean_output=off  mode=Lower Bit Location + Width  bit1=0  base1=MSB of Input  bit0=0  base0=LSB of Input  dbl_ovrd=off  block_type=slice
      settings: block_version=VER_STRING_GOES_HERE
  Slice4 : xbsIndex_r4/Slice  nbits=10  boolean_output=off  mode=Lower Bit Location + Width  bit1=0  base1=MSB of Input  bit0=0  base0=LSB of Input  dbl_ovrd=off  block_type=slice
      settings: block_version=VER_STRING_GOES_HERE
  AudioOut : Outport
  Amp : Outport  Port=2
  CmdToUser : Outport  Port=3
  Data2Archive : Outport  Port=4
  PhaseIncrement 8bits : Outport  Port=5
  NewCmdToUser : Outport  Port=6
  TX_Phase : Outport  Port=7
  NewValue : Outport  Port=8
  State : Outport  Port=9
  tag scope: DSPRAMrdbk=global
  wires:
  Convert4/1 -> PicoBlaze6/1
  Rst/1 -> Convert2/1
  PicoBlaze6/5 -> Convert3/1
  PicoBlaze6/4 -> Assert4/1, OutputRegister/2(PortId)
  PicoBlaze6/3 -> OutputRegister/1(Data)
  PicoBlaze6/1 -> Dual Port RAM/1
  Convert2/1 -> PicoBlaze6/5
  InputSelect/1(Out1) -> PicoBlaze6/2
  Dual Port RAM/1 -> Convert4/1
  Constant4/1 -> Dual Port RAM/3, Convert1/1
  Constant5/1 -> Dual Port RAM/2
  Slice2/1 -> InputSelect/1(Select)
  OutputRegister/1(Audio_Out) -> AudioOut/1
  AddrRam/1 -> Dual Port RAM/4
  OutputRegister/2(Amp) -> Amp/1
  DataRam/1 -> Dual Port RAM/5
  WriteRam/1 -> Dual Port RAM/6
  Convert1/1 -> PicoBlaze6/3, PicoBlaze6/4
  OutputRegister/3(Cmd2User) -> CmdToUser/1
  Strobe/1 -> InputSelect/3(strobe), Monostable2/1
  OutputRegister/6(Data2Archive) -> Dual Port RAM1/2, Data2Archive/1
  OutputRegister/7(PhaseIncrement) -> PhaseIncrement 8bits/1
  Cmd/1 -> Buffer/1(Cmd)
  Buffer/1(CmdOut) -> InputSelect/4(Cmd)
  OutputRegister/8(NewCmd) -> NewCmdToUser/1
  NewCmd/1 -> Buffer/2(NewCmd)
  OutputRegister/9(Ack_Fifo) -> Buffer/3(AckFifo)
  Mult/1 -> Slice1/1
  Slice1/1 -> InputSelect/5(MultOut)
  OutputRegister/4(Coeff) -> Reinterpret/1
  OutputRegister/5(Signal) -> Reinterpret1/1
  Convert3/1 -> OutputRegister/3(Write)
  BTauidioIN/1 -> InputSelect/6(BTaudioIN)
  [TX_High] -> Convert/1
  Convert/1 -> Mult/3
  Reinterpret/1 -> Mult/1
  Reinterpret1/1 -> Mult/2
  [Address] -> Slice4/1
  [RAMData] -> Dual Port RAM1/5
  Monostable1/1 -> Dual Port RAM1/6
  Dual Port RAM1/2 -> [DSPRAMrdbk]
  OutputRegister/10(RAMaddress) -> Dual Port RAM1/1
  OutputRegister/11(WriteRAM) -> Dual Port RAM1/3
  [WriteDSP_RAM] -> Monostable1/1
  Dual Port RAM1/1 -> InputSelect/7(RAMdata)
  Constant1/1 -> Concat/1
  [DSP2UserFIFOfull] -> Concat/3
  Concat/1 -> InputSelect/8(Status)
  OutputRegister/12(TXphase) -> TX_Phase/1
  [NoBTsignal] -> Concat/2
  OutputRegister/13(NewValue) -> NewValue/1
  FilterredSignal/1 -> Delay/1
  Monostable2/1 -> Convert5/1
  Convert5/1 -> Delay/2
  Delay/1 -> InputSelect/2(Signal)
  OutputRegister/14(State) -> State/1
  Assert4/1 -> Slice2/1
  PicoBlaze6/2 -> Assert1/1
  Slice4/1 -> Dual Port RAM1/4
  Assert1/1 -> Convert6/1
  Convert6/1 -> Dual Port RAM/7

== system N3_TE0722A4/DemodulationSSB1 ==
  note: (512kHz for 8kHz)
  note: Integration of 8 FIR streams
  note: Select I or Q part of the LO LUT
  note: 30364 with 49.152MHz clock and 8kHz sampling
      | BUT 30022 (7546 hex) with only 1kHz offset ie 87.956
      | or 45032 for 32.768MHz
      | or 30037 ($7555) for 88kHz
      | 45056 for 32.768MHz
      | 341 (0155 hex) for audio filterring - or 512 with 32.768MHz
  note: Pulses at twice carrier frequency
  note: Needs to run at fpgaclk!
  note: This is a 8kHz Square wave
  note: Set Frequency should be 839 for audio in
  note: This filter should be adjusted for 8kHz
  note: USES BLOCK RAM!
  note: Changed precission to fixed at output
  note: Reduced win amplitude to prevent saturation
  note: I
  note: Q
  note: I
  note: Q
  note: I+-Q
  SignalIn : Inport
  Trig : Inport  Port=2
  AGCandFilter1 : Subsystem
  Accumulator : xbsIndex_r4/Accumulator  operation=Add  n_bits=24  overflow=Wrap  scale=1  rst=off  hasbypass=on  infoeditControl=reset for floating point data type must be asserted for a minimum of 2 cycles  en=off  latency=0  msb_inp=100  msb=100  lsb=-100  use_behavioral_HDL=on  implementation=Fabric  dbl_ovrd=off  block_type=accum
      settings: xl_area=[9 18 0 18 0 0 0]  block_version=8.2.02
  AddSub : xbsIndex_r4/AddSub  mode=Addition or Subtraction  use_carryin=off  use_carryout=off  en=off  latency=0  precision=User Defined  arith_type="Signed  (2's comp)"  n_bits=18  bin_pt=17  quantization=Truncate  overflow=Wrap  use_behavioral_HDL=off  hw_selection=Fabric  pipelined=off  dbl_ovrd=off  block_type=addsub
      settings: block_version=12.2
  Baseband : xbsIndex_r4/Constant  const=512  gui_display_data_type=Fixed-point  arith_type=Unsigned  n_bits=16  bin_pt=0  preci_type=Single  exp_width=8  frac_width=24  explicit_period=off  period=1  equ=P=C  opselect=C  inp2=PCIN>>17  opr=+  inp1=P  carry=CIN  dbl_ovrd=off  block_type=constant
  CMult : xbsIndex_r4/CMult  const=1/sqrt(2)  gui_display_data_type=Fixed-point  const_n_bits=16  const_bin_pt=15  float_type=Single  exp_bits=8  fraction_bits=24  en=off  latency=1  precision=User Defined  arith_type="Signed  (2's comp)"  n_bits=18  bin_pt=17  quantization=Truncate  overflow=Wrap  use_behavioral_HDL=off  mem_type=Distributed RAM  pipeline=off  dbl_ovrd=off  block_type=cmult
      settings: block_version=12.2
  Concat : xbsIndex_r4/Concat  num_inputs=2  dbl_ovrd=off  block_type=concat
      settings: block_version=8.2.02
  Concat1 : xbsIndex_r4/Concat  num_inputs=2  dbl_ovrd=off  block_type=concat
      settings: block_version=8.2.02
  Concat2 : xbsIndex_r4/Concat  num_inputs=2  dbl_ovrd=off  block_type=concat
      settings: block_version=8.2.02
  Convert : xbsIndex_r4/Convert  gui_display_data_type=Fixed-point  arith_type=Unsigned  n_bits=1  bin_pt=0  float_type=Single  exp_bits=8  fraction_bits=24  quantization=Truncate  overflow=Wrap  en=off  latency=0  pipeline=off  dbl_ovrd=off  block_type=convert
  CtrlBitSequenceAddress : Subsystem
  CtrlSequencer : Subsystem
  Delay : xbsIndex_r4/Delay  rst=off  infoeditControl=Selection of Reset will increase slice count due to use of real FFs and instead of SRLs  en=off  latency=1  reg_retiming=off  dbl_ovrd=off  block_type=delay
      settings: block_version=12.2
  Delay1 : xbsIndex_r4/Delay  rst=off  infoeditControl=Selection of Reset will increase slice count due to use of real FFs and instead of SRLs  en=off  latency=1  reg_retiming=off  dbl_ovrd=off  block_type=delay
      settings: block_version=12.2
  FilterStreamIntegration : Subsystem
  LUT : xbsIndex_r4/ROM  depth=1024  initVector=[sin([0:255]*2*pi/256),-cos([0:255]*2*pi/256),win]*0.999  distributed_mem=Block RAM  rst=off  init_reg=0  en=off  latency=1  gui_display_data_type=Fixed-point  arith_type="Signed  (2's comp)"  n_bits=18  bin_pt=17  preci_type=Single  exp_width=8  frac_width=24  optimize=Area  use_rpm=on  dbl_ovrd=off  block_type=sprom
      settings: xl_area=[0 0 5 0 0 0 0]  block_version=8.2.02
  M1 : xbsIndex_r4/Mux  inputs=2  en=off  latency=1  precision=Full  arith_type=Unsigned  n_bits=16  bin_pt=14  quantization=Truncate  overflow=Wrap  dbl_ovrd=off  block_type=mux
      settings: xl_area=[5 9 0 9 0 0 0]  block_version=8.2.02
  M2 : xbsIndex_r4/Mux  inputs=4  en=off  latency=1  precision=Full  arith_type=Unsigned  n_bits=16  bin_pt=14  quantization=Truncate  overflow=Wrap  dbl_ovrd=off  block_type=mux
      settings: xl_area=[18 18 0 36 0 0 0]  block_version=8.2.02
  Monostable : MyFunctions/Monostable
  Mult : xbsIndex_r4/Mult  precision=User Defined  arith_type="Signed  (2's comp)"  n_bits=18  bin_pt=17  quantization=Truncate  overflow=Wrap  en=off  latency=2  use_behavioral_HDL=off  opt=Speed  use_embedded=on  optimum_pipeline=off  pipeline=on  dbl_ovrd=off  use_rpm=on  placement_style=Rectangular shape  block_type=mult
      settings: xl_area=[9 18 0 18 0 1 0]  block_version=8.2.02
  Mux : xbsIndex_r4/Mux  inputs=2  en=off  latency=0  precision=Full  arith_type=Unsigned  n_bits=16  bin_pt=14  quantization=Truncate  overflow=Wrap  dbl_ovrd=off  block_type=mux
  Register{,1..4} (5 alike) : xbsIndex_r4/Register  init=0  rst=off  en=on  dbl_ovrd=off  block_type=register
      settings: xl_area=[9 18 0 0 0 0 0]  block_version=8.2.02
  Reinterpret : xbsIndex_r4/Reinterpret  force_arith_type=on  arith_type="Signed  (2's comp)"  force_bin_pt=on  bin_pt=15  block_type=reinterpret
      settings: infoedit="Changes signal type without altering the binary representation.   You can changed the signal between signed and unsigned, and relocate the binary point.<br><br>Hardware notes: In hardware this block costs nothing.<br><br>Example:  Suppose the input is 6 bits wide, signed, with 2 fractional bits, and the output is forced to unsigned with 0 fractional bits.  Then an input of -2.0 (1110.00 in binary 2's complement) becomes an output of 56 (111000 in binary)."  block_version=8.2.02
  Slice : xbsIndex_r4/Slice  nbits=8  boolean_output=off  mode=Upper Bit Location + Width  bit1=0  base1=MSB of Input  bit0=0  base0=LSB of Input  dbl_ovrd=off  block_type=slice
      settings: block_version=8.2.02
  StreamControl1 : Subsystem
  DemodSignal : Outport
  DemodSqStrobe : Outport  Port=2
  wires:
  M2/1 -> Mult/1
  Mult/1 -> Register/1, Register2/1, Register1/1, CMult/1
  Register/1 -> M2/3
  Register1/1 -> M2/4
  Concat/1 -> M1/3
  CtrlSequencer/2(M2) -> M2/1
  CtrlSequencer/1(M1) -> Concat2/1, M1/1
  Accumulator/1 -> Slice/1
  Mux/1 -> Accumulator/1
  Concat1/1 -> M1/2
  SignalIn/1 -> Reinterpret/1
  Register2/1 -> FilterStreamIntegration/3(Signal)
  Trig/1 -> CtrlBitSequenceAddress/1(Trig), StreamControl1/1(Trig)
  CtrlSequencer/8(IncrmntStreamAddress) -> StreamControl1/2(IncStream)
  CtrlSequencer/6(LatchDemod) -> Register2/2
  CtrlSequencer/5(LatchQ) -> Register1/2, Delay1/1
  CtrlSequencer/4(LatchI) -> Register/2, Delay/1
  M1/1 -> Concat2/2
  CtrlSequencer/3(IQaddress) -> Concat1/1
  Concat2/1 -> LUT/1
  Slice/1 -> Concat1/2
  CtrlBitSequenceAddress/1(CtrlSequencerAddress) -> CtrlSequencer/1(In1)
  StreamControl1/1(LUT6LSBs) -> Concat/2
  StreamControl1/2(LUTwindow3MSBs) -> Concat/1
  StreamControl1/3(StreamAddress) -> FilterStreamIntegration/1(Stream2Accu)
  StreamControl1/4(StreamReachingMaturity) -> FilterStreamIntegration/5(StreamMaturing)
  StreamControl1/5(StreamReachingMaturityTrig) -> FilterStreamIntegration/4(Rst)
  CtrlSequencer/7(Accu) -> FilterStreamIntegration/2(Accu)
  Reinterpret/1 -> M2/2
  LUT/1 -> Mult/2
  StreamControl1/6(Square8kHz) -> DemodSqStrobe/1, Monostable/1
  AddSub/1 -> M2/5
  CtrlSequencer/10(IQadd_sub) -> AddSub/3
  CMult/1 -> Register3/1, Register4/1
  Delay/1 -> Register3/2
  Delay1/1 -> Register4/2
  Register3/1 -> AddSub/1
  Register4/1 -> AddSub/2
  [TX_High] -> Convert/1
  Convert/1 -> Mux/1
  [RXFreq] -> Mux/2
  Baseband/1 -> Mux/3
  FilterStreamIntegration/1(DemodSignal) -> AGCandFilter1/1(In1)
  Monostable/1 -> AGCandFilter1/2(AudioSampleClk)
  AGCandFilter1/1(Out1) -> DemodSignal/1

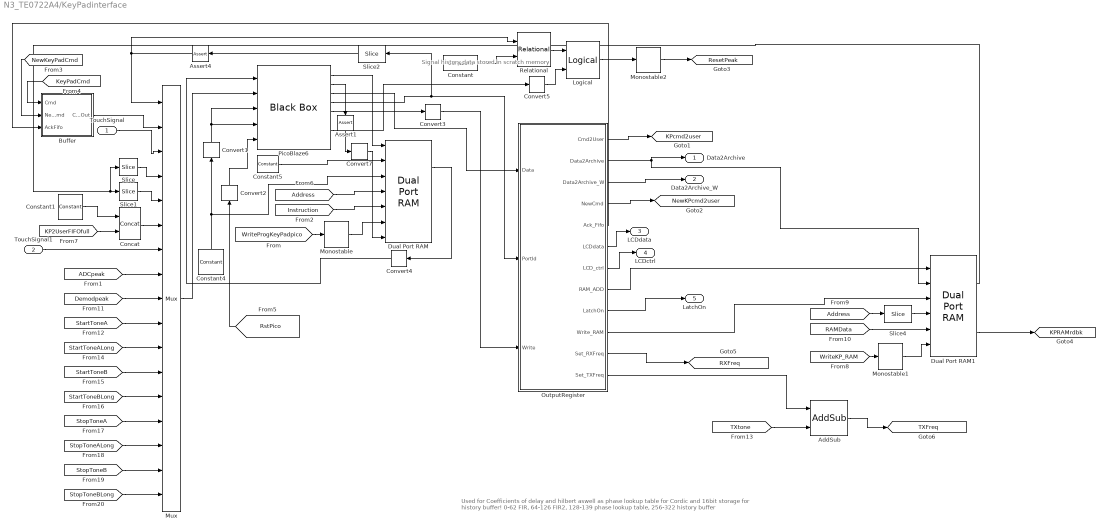
== system N3_TE0722A4/KeyPadinterface ==
  note: Used for Coefficients of delay and hilbert aswell as phase lookup table for Cordic and 16bit storage for history buffer!
      | 0-62 FIR, 64-126 FIR2, 128-139 phase lookup table, 256-322 history buffer
  note: Signal history data stored in scratch memory
  TouchSignal : Inport
  TouchSignal1 : Inport  Port=2
  AddSub : xbsIndex_r4/AddSub  mode=Addition  use_carryin=off  use_carryout=off  en=off  latency=0  precision=User Defined  arith_type=Unsigned  n_bits=16  bin_pt=0  quantization=Truncate  overflow=Wrap  use_behavioral_HDL=off  hw_selection=Fabric  pipelined=off  dbl_ovrd=off  block_type=addsub
  Assert1 : xbsIndex_r4/Assert  assert_type=off  type_source=Explicitly  gui_display_data_type=Fixed-point  arith_type="Signed  (2's comp)"  n_bits=16  bin_pt=14  preci_type=Single  exp_width=8  frac_width=24  assert_rate=on  rate_source=Explicitly  period=fpgaclk  output_port=on  block_type=assert
  Assert4 : xbsIndex_r4/Assert  assert_type=off  type_source=Explicitly  gui_display_data_type=Fixed-point  arith_type="Signed  (2's comp)"  n_bits=16  bin_pt=14  preci_type=Single  exp_width=8  frac_width=24  assert_rate=on  rate_source=Explicitly  period=fpgaclk  output_port=on  block_type=assert
  Buffer : Subsystem
  Concat : xbsIndex_r4/Concat  num_inputs=2  dbl_ovrd=off  block_type=concat
      settings: block_version=12.2
  Constant : xbsIndex_r4/Constant  const=7  gui_display_data_type=Fixed-point  arith_type=Unsigned  n_bits=4  bin_pt=0  preci_type=Single  exp_width=8  frac_width=24  explicit_period=off  period=1  equ=P=C  opselect=C  inp2=PCIN>>17  opr=+  inp1=P  carry=CIN  dbl_ovrd=off  block_type=constant
  Constant1 : xbsIndex_r4/Constant  const=0  gui_display_data_type=Fixed-point  arith_type=Unsigned  n_bits=7  bin_pt=0  preci_type=Single  exp_width=8  frac_width=24  explicit_period=on  period=fpgaclk  equ=P=C  opselect=C  inp2=PCIN>>17  opr=+  inp1=P  carry=CIN  dbl_ovrd=off  block_type=constant
      settings: block_version=VER_STRING_GOES_HERE
  Constant4 : xbsIndex_r4/Constant  const=0  gui_display_data_type=Fixed-point  arith_type=Boolean  n_bits=1  bin_pt=0  preci_type=Single  exp_width=8  frac_width=24  explicit_period=on  period=fpgaclk  equ=P=C  opselect=C  inp2=PCIN>>17  opr=+  inp1=P  carry=CIN  dbl_ovrd=off  block_type=constant
      settings: block_version=VER_STRING_GOES_HERE
  Constant5 : xbsIndex_r4/Constant  const=0  gui_display_data_type=Fixed-point  arith_type=Unsigned  n_bits=18  bin_pt=0  preci_type=Single  exp_width=8  frac_width=24  explicit_period=on  period=fpgaclk  equ=P=C  opselect=C  inp2=PCIN>>17  opr=+  inp1=P  carry=CIN  dbl_ovrd=off  block_type=constant
      settings: block_version=VER_STRING_GOES_HERE
  Convert{1..3,7} (4 alike) : xbsIndex_r4/Convert  gui_display_data_type=Fixed-point  arith_type=Boolean  n_bits=16  bin_pt=0  float_type=Single  exp_bits=8  fraction_bits=24  quantization=Truncate  overflow=Wrap  en=off  latency=0  pipeline=off  dbl_ovrd=off  block_type=convert
      Convert1 settings: xl_area=[0 0 0 0 0 0 0]  block_version=VER_STRING_GOES_HERE
      Convert2 settings: xl_area=[0, 0, 0, 0, 0, 0, 0]  block_version=VER_STRING_GOES_HERE
      Convert3 settings: xl_area=[0 0 0 0 0 0 0]  block_version=VER_STRING_GOES_HERE
      Convert7 settings: xl_area=[0, 0, 0, 0, 0, 0, 0]  block_version=VER_STRING_GOES_HERE
  Convert4 : xbsIndex_r4/Convert  gui_display_data_type=Fixed-point  arith_type=Unsigned  n_bits=18  bin_pt=0  float_type=Single  exp_bits=8  fraction_bits=24  quantization=Truncate  overflow=Wrap  en=off  latency=0  pipeline=off  dbl_ovrd=off  block_type=convert
      settings: xl_area=[0, 0, 0, 0, 0, 0, 0]  block_version=VER_STRING_GOES_HERE
  Convert5 : xbsIndex_r4/Convert  gui_display_data_type=Boolean  arith_type=Boolean  n_bits=16  bin_pt=0  float_type=Single  exp_bits=8  fraction_bits=24  quantization=Truncate  overflow=Wrap  en=off  latency=0  pipeline=off  dbl_ovrd=off  block_type=convert
      settings: xl_area=[0 0 0 0 0 0 0]  block_version=VER_STRING_GOES_HERE
  Dual Port RAM : xbsIndex_r4/Dual Port RAM  depth=1024*4  initVector=KeyPadprog  distributed_mem=Block RAM  init_a=0  init_b=0  rst_a=off  rst_b=off  en_a=on  en_b=off  latency=1  write_mode_A=Read After Write  write_mode_B=Read After Write  optimize=Area  dbl_ovrd=off  block_type=dpram
      settings: block_version=8.2.02
  Dual Port RAM1 : xbsIndex_r4/Dual Port RAM  depth=1024  initVector=KeyPadText  distributed_mem=Block RAM  init_a=0  init_b=0  rst_a=off  rst_b=off  en_a=off  en_b=off  latency=1  write_mode_A=Read After Write  write_mode_B=Read After Write  optimize=Area  dbl_ovrd=off  block_type=dpram
      settings: block_version=8.2.02
  Logical : xbsIndex_r4/Logical  logical_function=AND  inputs=2  en=off  latency=3  precision=Full  arith_type=Unsigned  n_bits=16  bin_pt=0  align_bp=on  dbl_ovrd=off  block_type=logical
  Monostable : MyFunctions/Monostable
  Monostable1 : MyFunctions/Monostable
  Monostable2 : MyFunctions/Monostable
  Mux : xbsIndex_r4/Mux  inputs=16  en=off  latency=1  precision=Full  arith_type=Unsigned  n_bits=16  bin_pt=14  quantization=Truncate  overflow=Wrap  dbl_ovrd=off  block_type=mux
      settings: xl_area=[16 0 0 32 0 0 0]  block_version=VER_STRING_GOES_HERE
  OutputRegister : Subsystem
  PicoBlaze6 : xbsIndex_r4/Black Box  init_code=kcpsm6_CE_256_4k_config  sim_method=Inactive  verbose=off  block_type=blackbox2
  Relational : xbsIndex_r4/Relational  mode=a=b  op_type=Bool  en=off  latency=0  dbl_ovrd=off  block_type=relational
  Slice : xbsIndex_r4/Slice  nbits=8  boolean_output=off  mode=Lower Bit Location + Width  bit1=0  base1=MSB of Input  bit0=0  base0=LSB of Input  dbl_ovrd=off  block_type=slice
      settings: block_version=8.2.02
  Slice1 : xbsIndex_r4/Slice  nbits=8  boolean_output=off  mode=Lower Bit Location + Width  bit1=0  base1=MSB of Input  bit0=8  base0=LSB of Input  dbl_ovrd=off  block_type=slice
      settings: block_version=8.2.02
  Slice2 : xbsIndex_r4/Slice  nbits=4  boolean_output=off  mode=Lower Bit Location + Width  bit1=0  base1=MSB of Input  bit0=0  base0=LSB of Input  dbl_ovrd=off  block_type=slice
      settings: block_version=VER_STRING_GOES_HERE
  Slice4 : xbsIndex_r4/Slice  nbits=10  boolean_output=off  mode=Lower Bit Location + Width  bit1=0  base1=MSB of Input  bit0=0  base0=LSB of Input  dbl_ovrd=off  block_type=slice
      settings: block_version=VER_STRING_GOES_HERE
  Data2Archive : Outport
  Data2Archive_W : Outport  Port=2
  LCDdata : Outport  Port=3
  LCDctrl : Outport  Port=4
  LatchOn : Outport  Port=5
  tag scope: KPRAMrdbk=global, KPcmd2user=global, NewKPcmd2user=global, RXFreq=global, ResetPeak=global, TXFreq=global
  wires:
  Convert4/1 -> PicoBlaze6/1
  [RstPico] -> Convert2/1
  PicoBlaze6/4 -> Slice2/1, OutputRegister/2(PortId)
  PicoBlaze6/3 -> OutputRegister/1(Data)
  Convert2/1 -> PicoBlaze6/5
  Mux/1 -> PicoBlaze6/2
  Dual Port RAM/1 -> Convert4/1
  Constant4/1 -> Dual Port RAM/3, Convert1/1
  Constant5/1 -> Dual Port RAM/2
  Slice2/1 -> Assert4/1
  Convert1/1 -> PicoBlaze6/3, PicoBlaze6/4
  OutputRegister/1(Cmd2User) -> [KPcmd2user]
  OutputRegister/2(Data2Archive) -> Data2Archive/1, Dual Port RAM1/2
  OutputRegister/4(NewCmd) -> [NewKPcmd2user]
  [NewKeyPadCmd] -> Buffer/2(NewCmd)
  OutputRegister/5(Ack_Fifo) -> Buffer/3(AckFifo)
  Convert3/1 -> OutputRegister/3(Write)
  Buffer/1(CmdOut) -> Mux/2
  [Instruction] -> Dual Port RAM/5
  TouchSignal/1 -> Mux/3
  OutputRegister/6(LCDdata) -> LCDdata/1
  OutputRegister/7(LCD_ctrl) -> LCDctrl/1
  [KeyPadCmd] -> Buffer/1(Cmd)
  Slice1/1 -> Mux/5
  OutputRegister/3(Data2Archive_W) -> Data2Archive_W/1
  OutputRegister/9(LatchOn) -> LatchOn/1
  [Address] -> Slice4/1
  [RAMData] -> Dual Port RAM1/5
  Monostable1/1 -> Dual Port RAM1/6
  [WriteKP_RAM] -> Monostable1/1
  Dual Port RAM1/2 -> [KPRAMrdbk]
  [Address] -> Dual Port RAM/4
  [WriteProgKeyPadpico] -> Monostable/1
  Monostable/1 -> Dual Port RAM/6
  OutputRegister/8(RAM_ADD) -> Dual Port RAM1/1
  OutputRegister/10(Write_RAM) -> Dual Port RAM1/3
  Dual Port RAM1/1 -> Slice/1, Slice1/1
  Concat/1 -> Mux/6
  Constant1/1 -> Concat/1
  TouchSignal1/1 -> Mux/7
  [KP2UserFIFOfull] -> Concat/2
  [ADCpeak] -> Mux/8
  [Demodpeak] -> Mux/9
  Constant/1 -> Relational/2
  Monostable2/1 -> [ResetPeak]
  [StartToneA] -> Mux/10
  OutputRegister/11(Set_RXFreq) -> [RXFreq]
  Relational/1 -> Logical/1
  PicoBlaze6/7 -> Convert5/1
  Logical/1 -> Monostable2/1
  Convert5/1 -> Logical/2
  OutputRegister/12(Set_TXFreq) -> AddSub/1
  [TXtone] -> AddSub/2
  AddSub/1 -> [TXFreq]
  Slice/1 -> Mux/4
  [StartToneALong] -> Mux/11
  [StartToneB] -> Mux/12
  [StartToneBLong] -> Mux/13
  [StopToneA] -> Mux/14
  [StopToneALong] -> Mux/15
  [StopToneB] -> Mux/16
  [StopToneBLong] -> Mux/17
  Slice4/1 -> Dual Port RAM1/4
  Assert4/1 -> Mux/1, Relational/1
  PicoBlaze6/1 -> Dual Port RAM/1
  PicoBlaze6/2 -> Assert1/1
  PicoBlaze6/5 -> Convert3/1
  Convert7/1 -> Dual Port RAM/7
  Assert1/1 -> Convert7/1
